simulink model "lademanagementsimulation"  (R2021b)
settings: Solver=VariableStepAuto  StartTime=0.0  StopTime=20  RelTol=1e-3
undefined symbols (not defined in the file): anzahlKunden, energieMaxAkku, ladezustandStart, solarPeakLeistung
libraries: SignalEditorBlockLib x1
settings Model: Creator=weber  LastModifiedBy=weber

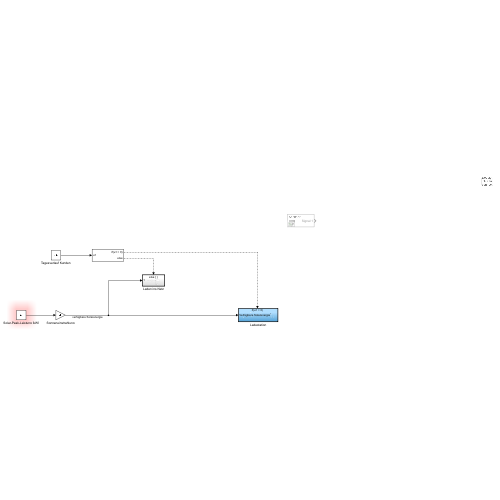
[thumbnail: Simulink's stored preview of the top-level diagram]
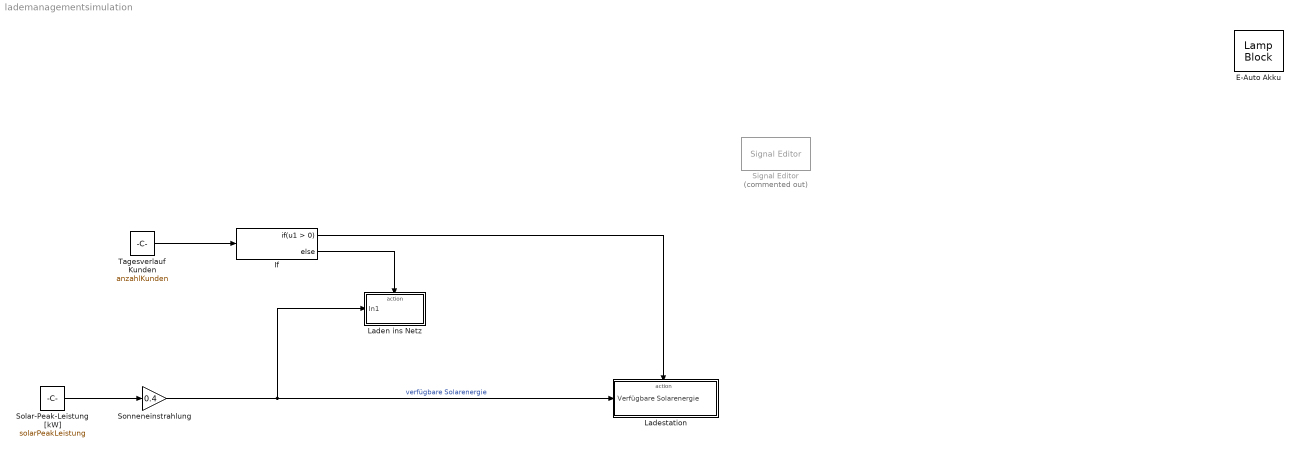
== system lademanagementsimulation ==
  E-Auto Akku : LampBlock  LabelPosition=Hide  Icon=Battery
  If : If
  Laden ins Netz : Subsystem  TreatAsAtomicUnit=on
  Ladestation : Subsystem  TreatAsAtomicUnit=on
  Signal Editor : SignalEditorBlockLib/Signal Editor  Commented=on  FileName=untitled.mat  ActiveScenario=Scenario  ActiveSignal=Signal 1  IsBus=off  OutputBusObjectStr=Bus: BusObject  SampleTime=0  Interpolate=off  ZeroCross=off  OutputAfterFinalValue=Setting to zero  Unit=inherit  PreserveSignalName=on
  Solar-Peak-Leistung [kW] : Constant  Value=solarPeakLeistung
  Sonneneinstrahlung : Gain  Gain=0.4
  Tagesverlauf Kunden : Constant  Value=anzahlKunden
  wires:
  Tagesverlauf Kunden/1 -> If/1
  Solar-Peak-Leistung [kW]/1 -> Sonneneinstrahlung/1
  If/2 -> Laden ins Netz/Action
  If/1 -> Ladestation/Action
  Sonneneinstrahlung/1 -> Laden ins Netz/1(In1), Ladestation/1(Verfügbare Solarenergie)  "verfügbare Solarenergie"

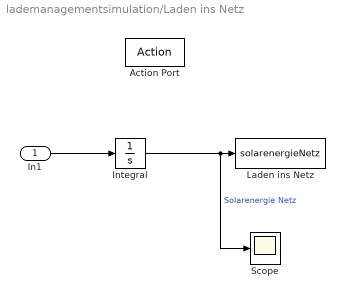
== system lademanagementsimulation/Laden ins Netz ==
  In1 : Inport
  Action Port : ActionPort  ActionPortLabel=else
  Integral : Integrator
  Laden ins Netz : ToWorkspace  VariableName=solarenergieNetz  SaveFormat=Timeseries  SampleTime=-1
  Scope : Scope
  wires:
  In1/1 -> Integral/1
  Integral/1 -> Scope/1, Laden ins Netz/1  "Solarenergie Netz"

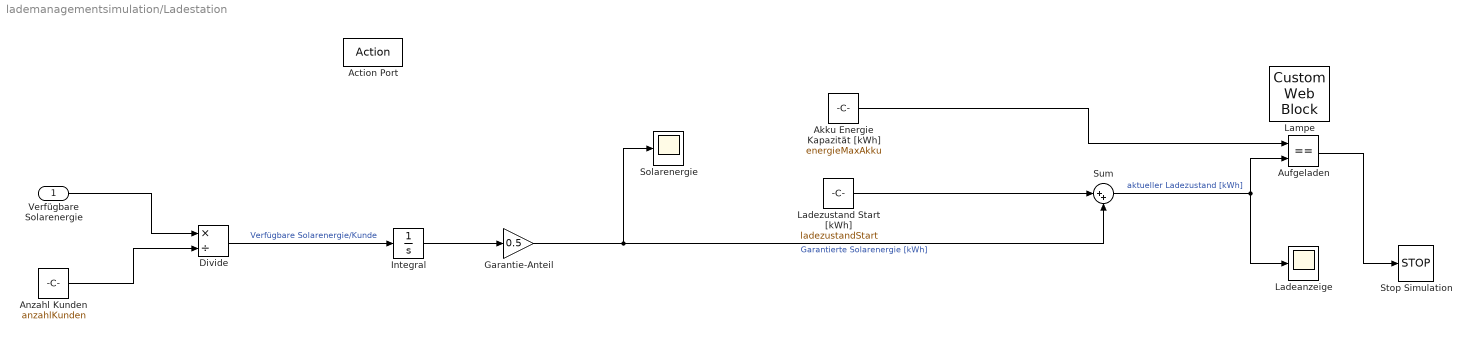
== system lademanagementsimulation/Ladestation ==
  Verfügbare Solarenergie : Inport
  Action Port : ActionPort  ActionPortLabel=if(u1 > 0)
  Akku Energie Kapazität [kWh] : Constant  Value=energieMaxAkku
  Anzahl Kunden : Constant  Value=anzahlKunden
  Aufgeladen : RelationalOperator  Operator===  OutDataTypeStr=boolean  RndMeth=Simplest
  Divide : Product  Inputs=*/
  Garantie-Anteil : Gain  Gain=0.5
  Integral : Integrator
  Ladeanzeige : Scope
  Ladezustand Start [kWh] : Constant  Value=ladezustandStart
  Lampe : CustomWebBlock  LabelPosition=Bottom  ShowInitialText=on  Configuration="{\"components\":[{\"name\":\"BackgroundImageComponent\",\"settings\":{\"image\":{\"size\":[150,150],\"src\":\"data:image\\/svg+xml;base64,PHN2ZyB4bWxucz0iaHR0cDovL3d3dy53My5vcmcvMjAwMC9zdmciIHhtbG5zOnhsaW5rPSJodHRwOi8vd3d3LnczLm9yZy8xOTk5L3hsaW5rIiB2aWV3Qm94PSIwIDAgNTAwIDUwMCI+PGRlZnM+PHN0eWxlPi5he2ZpbGw6dXJsKCNhKTt9LmJ7ZmlsbDp1cmwoI2IpO30uY3tmaWxsOnVybCgjYyk7fTwvc3R5bGU+PHJhZGlhbEdyYWRpZW50IGlkPSJhIiBjeD0iMjgzLjg0IiBjeT0iLTQ2Ni4zNyIgcj0iMzc1Ljc1IiBncmFkaWVudFRyYW5zZm9ybT0ibWF0cml4KDEuMzksIDAsIDAsIC0xLjM5LCAtMTUzLjU2LCAtNjQ0LjA4KSIg ...(+2088 chars)\",\"srcOrientation\":\"Right\"},\"position\":[0,0,1,1],\"scaleMode\":\"0\"}},{\"name\":\"LampShapeComponent\",\"settings\":{\"customMask\":{\"size\":[135,150],\"src\":\"data:image\\/svg+xml;base64,PHN2ZyBpZD0iTGF5ZXJfMSIgZGF0YS1uYW1lPSJMYXllciAxIiB4bWxucz0iaHR0cDovL3d3dy53My5vcmcvMjAwMC9zdmciIHZpZXdCb3g9IjAgMCA0MTEgNDU4Ij48ZGVmcz48c3R5bGU+LmNscy0xe2ZpbGw6I2ZkZjhjMTt9LmNscy0ye2ZpbGw6I2ZlZTEwMDt9LmNscy0ze2ZpbGw6IzIzMWYyMDt9LmNscy00e2ZpbGw6I2EwOWY5Zjt9LmNscy00LC5jbHMtNSwuY2xzLTZ7c3Ryb2tlOiMyMzFmMjA7c3Ryb2tlLW1pdGVybGltaXQ6MTA7fS5jbHMtNXtmaWxsOiNmZmY7fS5jbHMtNntmaWxsOm5vbmU7fTwvc3R5bGU+PC9kZWZz ...(+5168 chars)\",\"srcOrientation\":\"Right\"},\"defaultColor\":[0.7254901960784313,0,0],\"mask\":{\"id\":-1,\"type\":\"custom\"},\"maskScale\":0.8,\"position\":[0.1,0.1,0.8,0.8],\"shapeId\":0,\"states\":[{\"color\":[0,0,0],\"value\":0},{\"color\":[0.13333333333333333,0.7098039215686275,0.45098039215686275],\"value\":1}],\"type\":\"intersect\"}},{\"name\":\"ForegroundImageComponent\",\"settings\":{\"image\":{\"size\":[150,150],\"src\":\"data:image\\/svg+xml;base64,PHN2ZyB4bWxucz0iaHR0cDovL3d3dy53My5vcmcvMjAwMC9zdmciIHhtbG5zOnhsaW5rPSJodHRwOi8vd3d3LnczLm9yZy8xOTk5L3hsaW5rIiB2aWV3Qm94PSIwIDAgNTAwIDUwMCI+PGRlZnM+PHN0eWxlPi5he2ZpbGw6dXJsKCNhKTt9PC9zdHlsZT48bGluZWFyR3JhZGllbnQgaWQ9ImEiIHgxPSIxNzMuMDUiIHkxPSItNjI3Ljc4IiB4Mj0iMTczLjA1IiB5Mj0iLTUyMi40MyIgZ3JhZGllbnRUcmFuc2Zvcm09Im1hdHJpeCgxLjI5LCAwLCAwLCAtMS4zMywgMjcuMTMsIC02MjguMzEpIiBncmFkaWVudFVuaXRzPSJ1c2VyU3BhY2VPblVzZSI+PHN0b3Agb2Zmc2V0PSIwIiBzdG9wLWNvbG9yPSIjZmZmIiBzdG9wLW9wYWNpdHk9IjAuMjUiLz48c3RvcCBvZmZzZXQ9IjEiIHN0b3AtY29sb3I9IiNmZmYiIHN0b3Atb3BhY2l0eT0iMCIvPjwvbGluZWFyR3JhZGllbnQ+PC9kZWZzPjxwYXRoIGNsYXNzPSJhIiBkPSJNNDI5LjMsMTkwLjY2QzQwMi40NSwxMTQuNTEsMzMyLjY3LDYwLjE3LDI1MC44NSw2MC4xN2MtODMuNDMsMC0xNTQuMjgsNTYuNDItMTc5Ljk1LDEzNSwxNS4zNCwzOSw4OC4xMSw3LDE3Ny4wNyw3QzM0MCwyMDIuMDgsNDE3LjI2LDIzNi40Niw0MjkuMywxOTAuNjZaIi8+PC9zdmc+\",\"srcOrientation\":\"Right\"},\"isForeground\":1,\"position\":[0,0,1,1],\"scaleMode\":\"0\"}}],\"settings\":{\"BindingType\":\"signal\",\"aspectRatio\":1.032258064516129,\"backgroundColor\":[0,0,0],\"backgroundOffset\":0.14,\"backgroundOpacity\":1,\"blockOrientation\":\"Right\",\"fixedAspectRatio\":\"on\",\"showBackgroundColor\":false,\"value\":0},\"type\":\"Lamp\"}"
  Solarenergie : Scope
  Stop Simulation : Stop
  Sum : Sum  Inputs=|++
  wires:
  Verfügbare Solarenergie/1 -> Divide/1
  Sum/1 -> Aufgeladen/2, Ladeanzeige/1  "aktueller Ladezustand [kWh]"
  Ladezustand Start [kWh]/1 -> Sum/1
  Akku Energie Kapazität [kWh]/1 -> Aufgeladen/1
  Aufgeladen/1 -> Stop Simulation/1
  Integral/1 -> Garantie-Anteil/1
  Divide/1 -> Integral/1  "Verfügbare Solarenergie/Kunde"
  Anzahl Kunden/1 -> Divide/2
  Garantie-Anteil/1 -> Sum/2, Solarenergie/1  "Garantierte Solarenergie [kWh]"
